simulink model "MODULATOR_DEMODULATOR"  (R2025b)
settings: Solver=VariableStepAuto  StartTime=0.0  StopTime=10.0  RelTol=1e-3
libraries: commdigbbndpm3 x2, commchan3 x1, commrandsrc3 x1
settings Model: Creator=Nandan Prasad  LastModifiedBy=Nandan Prasad

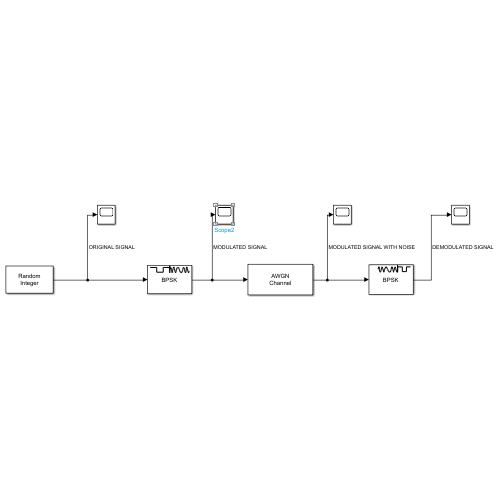
[thumbnail: Simulink's stored preview of the top-level diagram]
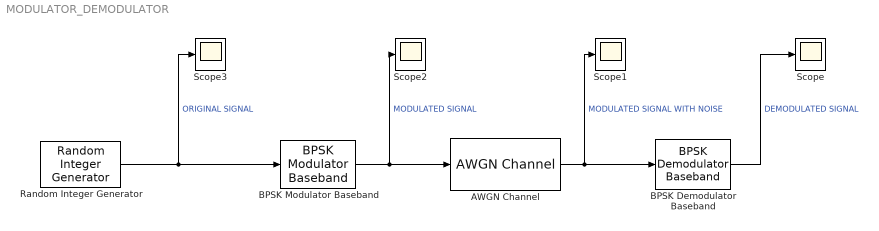
== system MODULATOR_DEMODULATOR ==
  AWGN Channel : commchan3/AWGN Channel  LegacyMode=off  NoiseMethod="Signal to noise ratio  (SNR)"  noiseMode="Signal to noise ratio  (SNR)"  EbNo=10  EsNo=10  SNR=10  BitsPerSymbol=1  SignalPower=1  SpecifySymbolPeriod=off  SamplesPerSymbol=1  SymbolPeriod=1  VarianceSource=Parameter  Variance=1  RandomStream=Global stream  Seed=67  SimulateUsing=Code generation
  BPSK Demodulator Baseband : commdigbbndpm3/BPSK Demodulator Baseband  DecType=Hard decision  VarSource=Dialog  Variance=1  Ph=0  outDtype=Inherit via internal rule  derotateFactorWordLen=16  derotateFactorDataTypeStr=Inherit: Same word length as input  derotateFactorLastDataTypeStr=Inherit: Same word length as input
      settings: LibrarySourceBlock=|
      | commhdldigbbndpm/BPSK
      | Demodulator
      | Baseband
  BPSK Modulator Baseband : commdigbbndpm3/BPSK Modulator Baseband  Ph=0  outDtype=double  outWordLen=16  outUDDataType=sfix(16)  outFracLenMode=Best precision  outFracLen=15  outDataTypeStr=double  outLastDataTypeStr=double
      settings: LibrarySourceBlock=|
      | commhdldigbbndpm/BPSK
      | Modulator
      | Baseband
  Random Integer Generator : commrandsrc3/Random Integer Generator  SetSize=2  SeedSource=Auto  Seed=0  SampleTime=1  SamplesPerFrame=1  OutputDataType=double  SimulateUsing=Interpreted execution
  Scope{,1..3} (4 alike) : Scope
      Scope2 settings: DataLoggingVariableName=ScopeData2
      Scope3 settings: DataLoggingVariableName=ScopeData3
  wires:
  Random Integer Generator/1 -> Scope3/1, BPSK Modulator Baseband/1  "ORIGINAL SIGNAL"
  BPSK Modulator Baseband/1 -> Scope2/1, AWGN Channel/1  "MODULATED SIGNAL"
  AWGN Channel/1 -> Scope1/1, BPSK Demodulator Baseband/1  "MODULATED SIGNAL WITH NOISE"
  BPSK Demodulator Baseband/1 -> Scope/1  "DEMODULATED SIGNAL"
